simulink model "EcoSIM3_P2_C2_WIP"  (R2014b)
settings: Solver=ode1  SolverMode=SingleTasking  StartTime=0.0  StopTime=4  FixedStep=0.01  RelTol=1e-3
PostLoadFcn:
  | %, if any(exist('dsrtsu_mdlpostloadfcn', 'file') == [2, 3, 6]), try dsrtsu_mdlpostloadfcn('Execute', bdroot); catch fprintf('Error in PostLoadFcn (dsrtsu_mdlpostloadfcn) for model "%s":\n %s\n', bdroot, lasterr); end, end,
InitFcn:
  | tic
  | %Startup_EcoSIM
undefined symbols (not defined in the file or in its folder): canChannel, Controls, DriveCycles, Driver, EM_EFF_MAP, EM_PwrLoss_MAP, EngPwr, EngSpd, EngTrq, Glbl, Overwritten_Mode, Plants, Power, sigbuilder_block, Torque, Trialmap, Veh_Dynamics
libraries: simulink x135, canmsglib x113, fl_lib x104, canlib x89, nesl_utility x56, sdl_lib x29, dspsigops x6, dspswit3 x5, dspstat3 x2, commnoisgen2 x1, dspfdesign x1
(part 2 of 21)

== system EcoSIM3_P2_C2_WIP/Powertrain/Vehicle Dynamics ==
  note: 0.34 - Dynamic Rolling radius that
      | Brandon has for Goodyear Eagle tyres
  note: Tyre diameter- If tyre dia is kept at dyno test value (original * 1.12), energy consumption
      | for drive cycles is low as motor speed decreases, but time taken to reach 60 mph
      | increases because road torque decreases
  note: Velocity of the vehicle in m/s
  note: VEHICLE DYNAMICS
  note: Negative Torque from brakes
  Beta : Inport
  " Front Right Tire" : sdl_lib/Tires & Vehicles/Tire (Magic Formula)  parameterization=1  F_z1=Plants.Front_wh.Rated_Vertical_Load N  F_x1=Plants.Front_wh.Rated_Peak_Long_Force N  kappa1=Plants.Front_wh.Tire.Slip_At_Peak_Force  B_m=10  C_m=1.9  D_m=1  E_m=0.97  fz0=4e+3 N  p_Cx=1.685  p_Dx=[ 1.21 -0.037 ]  p_Ex=[ 0.344 0.095 -0.02 0 ]  p_Kx=[ 21.51 -0.163 0.245 ]  p_Hx=[ -0.002 0.002 ]  p_Vx=[ 0 0 ]  v_tr_thr=Plants.Front_wh.Tire.Slip_Calculation_Velocity_Threshold m/s  r_e=Plants.Front_wh.Tire.rollrad m  model_compliance=0  stiffness=1e+6 N/m  damping=1000 N/(m/s)  model_inertia=1  inertia=Plants.Front_wh.Wheel_Inertia kg*m^2  initial_velocity=0 rpm  model_resistance=1  resistance_model=1  coeff=Plants.Front_wh.Tire.Constant_coeff  p_tire=250e3 Pa  alpha=-0.003  beta=0.97  coeff_a=84e-4  coeff_b=6.2e-4 s/m  coeff_c=1.6e-4 s^2/m^2  v_thr=Plants.Front_wh.Tire.Velocity_threshold m/s
  1-D Lookup Table : Lookup_n-D  NumberOfTableDimensions=1  BreakpointsForDimension1=Plants.Front_br.Brake_Beta_Cmd  Table=Plants.Front_br.Brake_Friction_Map  InternalRulePriority=Speed  RndMeth=Simplest  InputSameDT=on
  Double-Shoe Brake1 : sdl_lib/Brakes & Detents/Rotational/Double-Shoe Brake  r_drum=Plants.Front_br.Drum_radius mm  r_act=Plants.Front_br.Actuator_location mm  r_pin=Plants.Front_br.Pin_location_rad mm  theta_pin=Plants.Front_br.Pin_location_ang deg  theta_0=Plants.Front_br.Shoe_begin_ang deg  theta_shoe=Plants.Front_br.Shoe_span deg  mu_visc=Plants.Front_br.Viscous_fric_coeff N*m/(rad/s)  mu=Plants.Front_br.Contact_fric_coeff  w_thr=Plants.Front_br.Angular_vel_threshold rad/s
  Double-Shoe Brake2 : sdl_lib/Brakes & Detents/Rotational/Double-Shoe Brake  r_drum=Plants.Rear_br.Drum_radius mm  r_act=Plants.Rear_br.Actuator_location mm  r_pin=Plants.Rear_br.Pin_location_rad mm  theta_pin=Plants.Rear_br.Pin_location_ang deg  theta_0=Plants.Rear_br.Shoe_begin_ang deg  theta_shoe=Plants.Rear_br.Shoe_span deg  mu_visc=Plants.Rear_br.Viscous_fric_coeff N*m/(rad/s)  mu=Plants.Rear_br.Contact_fric_coeff  w_thr=Plants.Rear_br.Angular_vel_threshold rad/s
  Double-Shoe Brake3 : sdl_lib/Brakes & Detents/Rotational/Double-Shoe Brake  r_drum=Plants.Front_br.Drum_radius mm  r_act=Plants.Front_br.Actuator_location mm  r_pin=Plants.Front_br.Pin_location_rad mm  theta_pin=Plants.Front_br.Pin_location_ang deg  theta_0=Plants.Front_br.Shoe_begin_ang deg  theta_shoe=Plants.Front_br.Shoe_span deg  mu_visc=Plants.Front_br.Viscous_fric_coeff N*m/(rad/s)  mu=Plants.Front_br.Contact_fric_coeff  w_thr=Plants.Front_br.Angular_vel_threshold rad/s
  Double-Shoe Brake4 : sdl_lib/Brakes & Detents/Rotational/Double-Shoe Brake  r_drum=Plants.Rear_br.Drum_radius mm  r_act=Plants.Rear_br.Actuator_location mm  r_pin=Plants.Rear_br.Pin_location_rad mm  theta_pin=Plants.Rear_br.Pin_location_ang deg  theta_0=Plants.Rear_br.Shoe_begin_ang deg  theta_shoe=Plants.Rear_br.Shoe_span deg  mu_visc=Plants.Rear_br.Viscous_fric_coeff N*m/(rad/s)  mu=Plants.Rear_br.Contact_fric_coeff  w_thr=Plants.Rear_br.Angular_vel_threshold rad/s
  Front Brake Bias : fl_lib/Physical Signals/Functions/PS Gain  gain=Plants.Front_br.brake_F_propor
  Front Left Tire : sdl_lib/Tires & Vehicles/Tire (Magic Formula)  parameterization=1  F_z1=Plants.Front_wh.Rated_Vertical_Load N  F_x1=Plants.Front_wh.Rated_Peak_Long_Force N  kappa1=Plants.Front_wh.Tire.Slip_At_Peak_Force  B_m=10  C_m=1.9  D_m=1  E_m=0.97  fz0=4e+3 N  p_Cx=1.685  p_Dx=[ 1.21 -0.037 ]  p_Ex=[ 0.344 0.095 -0.02 0 ]  p_Kx=[ 21.51 -0.163 0.245 ]  p_Hx=[ -0.002 0.002 ]  p_Vx=[ 0 0 ]  v_tr_thr=Plants.Front_wh.Tire.Slip_Calculation_Velocity_Threshold m/s  r_e=Plants.Front_wh.Tire.rollrad m  model_compliance=0  stiffness=1e+6 N/m  damping=1000 N/(m/s)  model_inertia=1  inertia=Plants.Front_wh.Wheel_Inertia kg*m^2  initial_velocity=0 rpm  model_resistance=1  resistance_model=1  coeff=Plants.Front_wh.Tire.Constant_coeff  p_tire=250e3 Pa  alpha=-0.003  beta=0.97  coeff_a=84e-4  coeff_b=6.2e-4 s/m  coeff_c=1.6e-4 s^2/m^2  v_thr=Plants.Front_wh.Tire.Velocity_threshold m/s
  PS-Simulink Converter : nesl_utility/PS-Simulink Converter  PhysicalDomain=network_engine_domain  SubClassName=ps_output  LeftPortType=input  RightPortType=output  PseudoPeriodic=off  Frequencies=[]  Unit=1  AffineConversion=off
  PS-Simulink Converter1 : nesl_utility/PS-Simulink Converter  PhysicalDomain=network_engine_domain  SubClassName=ps_output  LeftPortType=input  RightPortType=output  PseudoPeriodic=off  Frequencies=[]  Unit=1  AffineConversion=off
  Rear Differential : sdl_lib/Gears/Differential  driveshaft_location=2  cd_ratio=Plants.Rear_Diff.Diff_ratio  friction_model=2  efficiency=Plants.Rear_Diff.Ordinary_efficiencies  mu_visc=Plants.Rear_Diff.damp N*m/(rad/s)  w_thr=Plants.Rear_Diff.Velocity_thresholds rad/s
  Rear Brake Bias : fl_lib/Physical Signals/Functions/PS Gain  gain=Plants.Rear_br.brake_R_propor
  Rear Right Tire : sdl_lib/Tires & Vehicles/Tire (Magic Formula)  parameterization=1  F_z1=Plants.Rear_wh.Rated_Vertical_Load N  F_x1=Plants.Rear_wh.Rated_Peak_Long_Force N  kappa1=Plants.Rear_wh.Tire.Slip_At_Peak_Force  B_m=10  C_m=1.9  D_m=1  E_m=0.97  fz0=4e+3 N  p_Cx=1.685  p_Dx=[ 1.21 -0.037 ]  p_Ex=[ 0.344 0.095 -0.02 0 ]  p_Kx=[ 21.51 -0.163 0.245 ]  p_Hx=[ -0.002 0.002 ]  p_Vx=[ 0 0 ]  v_tr_thr=Plants.Rear_wh.Tire.Slip_Calculation_Velocity_Threshold m/s  r_e=Plants.Front_wh.Tire.rollrad m  model_compliance=0  stiffness=1e+6 N/m  damping=1000 N/(m/s)  model_inertia=1  inertia=Plants.Rear_wh.Wheel_Inertia kg*m^2  initial_velocity=0 rpm  model_resistance=1  resistance_model=1  coeff=Plants.Rear_wh.Tire.Constant_coeff  p_tire=250e3 Pa  alpha=-0.003  beta=0.97  coeff_a=84e-4  coeff_b=6.2e-4 s/m  coeff_c=1.6e-4 s^2/m^2  v_thr=Plants.Rear_wh.Tire.Velocity_threshold m/s
  Rear Right Tires : sdl_lib/Tires & Vehicles/Tire (Magic Formula)  parameterization=1  F_z1=Plants.Rear_wh.Rated_Vertical_Load N  F_x1=Plants.Rear_wh.Rated_Peak_Long_Force N  kappa1=Plants.Rear_wh.Tire.Slip_At_Peak_Force  B_m=10  C_m=1.9  D_m=1  E_m=0.97  fz0=4e+3 N  p_Cx=1.685  p_Dx=[ 1.21 -0.037 ]  p_Ex=[ 0.344 0.095 -0.02 0 ]  p_Kx=[ 21.51 -0.163 0.245 ]  p_Hx=[ -0.002 0.002 ]  p_Vx=[ 0 0 ]  v_tr_thr=Plants.Rear_wh.Tire.Slip_Calculation_Velocity_Threshold m/s  r_e=Plants.Front_wh.Tire.rollrad m  model_compliance=0  stiffness=1e+6 N/m  damping=1000 N/(m/s)  model_inertia=1  inertia=Plants.Rear_wh.Wheel_Inertia kg*m^2  initial_velocity=0 rpm  model_resistance=1  resistance_model=1  coeff=Plants.Rear_wh.Tire.Constant_coeff  p_tire=250e3 Pa  alpha=-0.003  beta=0.97  coeff_a=84e-4  coeff_b=6.2e-4 s/m  coeff_c=1.6e-4 s^2/m^2  v_thr=Plants.Rear_wh.Tire.Velocity_threshold m/s
  Road Grade : fl_lib/Physical Signals/Sources/PS Constant  constant=0
  Scope1 : Scope  Commented=on  NumInputPorts=2
      settings: TimeRange=0.05746676406135975  YMin=-0.001119~-0.000858  YMax=-0.00111~-0.00084  SaveName=ScopeData11
  Sensor : Subsystem
  Simulink-PS Converter1 : nesl_utility/Simulink-PS Converter  PhysicalDomain=network_engine_domain  SubClassName=ps_input  LeftPortType=input  RightPortType=output  PseudoPeriodic=off  Frequencies=[]  NoiseDistribution=none  NoiseParameters=[]  Unit=N  AffineConversion=off  InputFiltering=off  SimscapeFilterOrder=1  InputFilterTimeConstant=0.001  UdotUserProvided=1
  Subsystem : Subsystem
  Vehicle Body : sdl_lib/Tires & Vehicles/Vehicle Body  mass=Veh_Dynamics.Body.Mass kg  n_w=2  x_f=Veh_Dynamics.Body.Distance_CG_FrontAxle m  x_r=Veh_Dynamics.Body.Distance_CG_RearAxle m  y_c=Veh_Dynamics.Body.Distance_CG_Ground m  area=Veh_Dynamics.Body.Frontal_Area m^2  Cd=Veh_Dynamics.Body.Aero_Drag_Coeff  v0=0 m/s  g=9.81 m/s^2  rho=1.18 kg/m^3
  Wind velocity : fl_lib/Physical Signals/Sources/PS Constant  constant=0
  MC_Coupler_Out : PMIOPort  Tag=PMCPort  Port=1  Side=Left
  Vehicle_Speed [m/s] : Outport
  wires:
  PS-Simulink Converter/1 -> Scope1/1  "LF_Wheel_Slip"
  PS-Simulink Converter1/1 -> Scope1/2  "LR_Wheel_Slip"
  Beta/1 -> 1-D Lookup Table/1
  1-D Lookup Table/1 -> Simulink-PS Converter1/1
  Sensor/1(Sensor_Out) -> Vehicle_Speed [m/s]/1
  connections:
  " Front Right Tire"/LConn1 -- Vehicle Body/RConn2 -- Front Left Tire/LConn1
  Rear Right Tire/LConn1 -- Vehicle Body/RConn1 -- Rear Right Tires/LConn1
  Sensor/RConn1 -- Rear Differential/RConn2 -- Rear Right Tires/LConn2 -- Double-Shoe Brake2/LConn2
  Rear Right Tire/LConn2 -- Double-Shoe Brake4/LConn2 -- Sensor/RConn2 -- Rear Differential/RConn1
  " Front Right Tire"/RConn2 -- Front Left Tire/RConn2 -- Subsystem/RConn1 -- Rear Right Tire/RConn2 -- Rear Right Tires/RConn2
  Rear Brake Bias/LConn1 -- Simulink-PS Converter1/RConn1 -- Front Brake Bias/LConn1
  Double-Shoe Brake3/LConn1 -- Double-Shoe Brake1/LConn1 -- Front Brake Bias/RConn1
  Front Left Tire/LConn2 -- Sensor/LConn3 -- " Front Right Tire"/LConn2 -- Sensor/LConn2 -- Double-Shoe Brake1/LConn2 -- Double-Shoe Brake3/LConn2
  Double-Shoe Brake2/LConn1 -- Rear Brake Bias/RConn1 -- Double-Shoe Brake4/LConn1
  Subsystem/LConn1 -- Vehicle Body/LConn1
  Road Grade/RConn1 -- Vehicle Body/RConn3
  PS-Simulink Converter1/LConn1 -- Rear Right Tires/RConn1
  PS-Simulink Converter/LConn1 -- " Front Right Tire"/RConn1
  Vehicle Body/LConn2 -- Sensor/LConn1
  MC_Coupler_Out/RConn1 -- Rear Differential/LConn1
  Vehicle Body/LConn3 -- Wind velocity/RConn1

== system EcoSIM3_P2_C2_WIP/RTI Data/RTI Data Store ==
  RTI Data Store : Subsystem  mask(RTI_DATA_STORE){}
      mask help:
      | RTI Data Store Block. This block is used by RTI to store internal model dependent data. Deleting this block will result in data loss.
      |
      | NEVER DELETE, COPY, OR MODIFY THIS BLOCK!
      mask Help:
      | RTI Data Store Block. This block is used by RTI to store internal model dependent data. Deleting this block will result in data loss.
      | 
      | NEVER DELETE, COPY, OR MODIFY THIS BLOCK!
      mask Display: text(0.5, 0.5, ' ', 'HorizontalAlignment', 'center');

== system EcoSIM3_P2_C2_WIP/Supervisory Controller/Charging Handshake ==
  In1 : Inport
  Bus Creator : BusCreator  Inputs=2
  Bus Selector1 : BusSelector  OutputSignals=From_GCM.GCM_CAN_Out.charge_mode_request,ESS_Transmit.ESS_Electrical_Out.chga_ena,ESS_Transmit.ESS_CAN_Out.BCM_Status.bcm_chg_done,ESS_Transmit.ESS_CAN_Out.BCM_Data2.bcm_balancing,ESS_Transmit.ESS_CAN_Out.BCM_Status.bcm_ready,ESS_Transmit.ESS_CAN_Out.BCM_Status.bcm_on_plug,ESS_Transmit.ESS_CAN_Out.BCM_Status.bcm_chgc_stat
  Chart1 : Stateflow chart  TreatAsAtomicUnit=on
  Compare To Constant : simulink/Logic and Bit Operations/Compare To Constant  relop===  const=1  OutDataTypeStr=boolean
  Constant1 : Constant  Value=0
  Data Type Conversion : DataTypeConversion
  Data Type Conversion1 : DataTypeConversion
  Terminator1 : Terminator
  Terminator3 : Terminator
  Out1 : Outport
  tag scope: Charging_Complete=global
  wires:
  Data Type Conversion1/1 -> Bus Creator/2  "PON"
  Data Type Conversion/1 -> Bus Creator/1  "chga_wake"
  Bus Selector1/1 -> Chart1/1(charge_mode_request)  "<charge_mode_request>"
  Bus Selector1/2 -> Chart1/2(chga_ena)  "<chga_ena>"
  Chart1/1(chga_wake) -> Data Type Conversion/1
  Chart1/2(PON) -> Data Type Conversion1/1
  Bus Creator/1 -> Out1/1
  In1/1 -> Bus Selector1/1
  Constant1/1 -> Chart1/4(bcm_balancing)
  Bus Selector1/3 -> Chart1/3(bcm_chg_done)  "<bcm_chg_done>"
  Bus Selector1/4 -> Terminator1/1  "<bcm_balancing>"
  Chart1/3(Charging_Complete) -> [Charging_Complete]
  Bus Selector1/5 -> Chart1/5(bcm_ready)  "<bcm_ready>"
  Bus Selector1/6 -> Chart1/6(bcm_on_plug)  "<bcm_on_plug>"
  Bus Selector1/7 -> Compare To Constant/1  "<bcm_chgc_stat>"
  Compare To Constant/1 -> Terminator3/1  "Charging_Light_On"

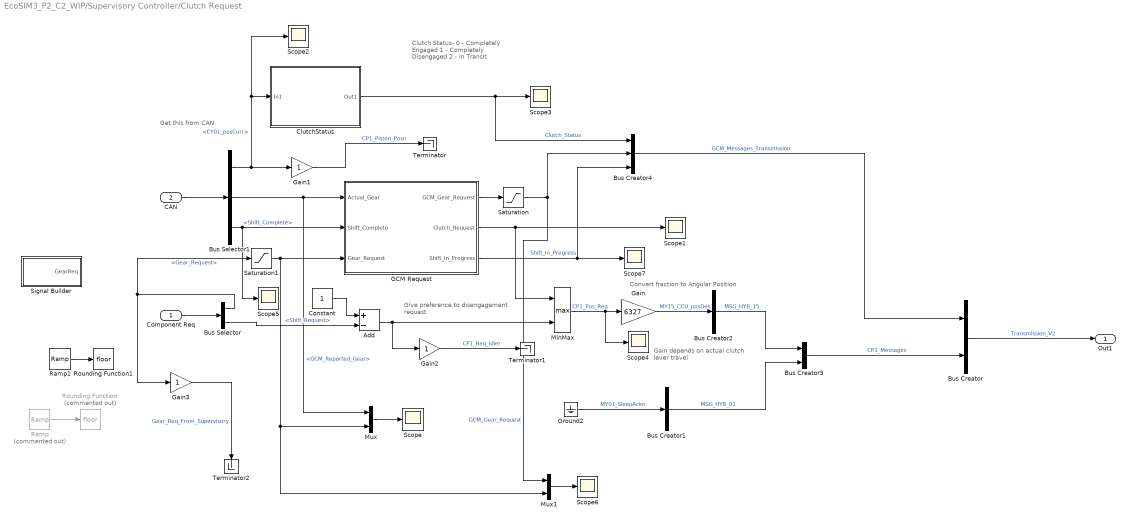
== system EcoSIM3_P2_C2_WIP/Supervisory Controller/Clutch Request ==
  note: Get this from CAN
  note: Convert fraction to Angular Position
  note: Clutch Status-
      | 0 - Completely Engaged
      | 1 - Completely Disengaged
      | 2 - In Transit
  note: Gain depends on actual
      | clutch lever travel
  note: Give preference to disengagement
      | request
  Component Req : Inport
  CAN : Inport  Port=2
  Add : Sum  Inputs=+-
  Bus Creator : BusCreator  Inputs=2
  Bus Creator1 : BusCreator  Inputs=1
  Bus Creator2 : BusCreator  Inputs=1
  Bus Creator3 : BusCreator  Inputs=2
  Bus Creator4 : BusCreator  Inputs=3
  Bus Selector : BusSelector  OutputSignals=Trans_Receive.Gear_Request,Trans_Receive.Shift_Request
  Bus Selector1 : BusSelector  OutputSignals=CP1_Transmit.CP1_CAN_Out.CCU_HYB_01.CY01_posCurr,From_GCM.GCM_CAN_Out.Shift_Status_to_MABx.GCM_Reported_Gear,From_GCM.GCM_CAN_Out.Shift_Status_to_MABx.Shift_Complete
  ClutchStatus : Subsystem
  Constant : Constant
  GCM Request : Stateflow chart  TreatAsAtomicUnit=on
  Gain : Gain  Gain=6327
  Gain1 : Gain
  Gain2 : Gain
  Gain3 : Gain
  Ground2 : Ground
  MinMax : MinMax  Function=max  Inputs=2
  Mux : Mux  Inputs=2
  Mux1 : Mux  Inputs=2
  Ramp : simulink/Sources/Ramp  Commented=on  slope=1  start=0  X0=1
  Ramp1 : simulink/Sources/Ramp  slope=0.5  start=0  X0=-1
  Rounding Function : Rounding  Commented=on
  Rounding Function1 : Rounding
  Saturation : Saturate  UpperLimit=5  LowerLimit=-1
  Saturation1 : Saturate  UpperLimit=5  LowerLimit=-1
  Scope{,1..7} (8 alike) : Scope
      Scope settings: YMin=0  SaveName=ScopeData20
      Scope1 settings: SaveName=ScopeData22
      Scope2 settings: YMin=0  YMax=8000  SaveName=ScopeData35
      Scope3 settings: YMin=0  YMax=8000  SaveName=ScopeData36
      Scope4 settings: SaveName=ScopeData37
      Scope5 settings: SaveName=ScopeData38
      Scope6 settings: SaveName=ScopeData45
      Scope7 settings: SaveName=ScopeData61
  Signal Builder : Subsystem  Tag=STV Subsys  LoadFcn=sigbuilder_block('load');  StartFcn=sigbuilder_block('start');  StopFcn=sigbuilder_block('stop');  ClipboardFcn=sigbuilder_block('clipboard');  mask(Sigbuilder block){}
      mask help: Simulink:masks:SigbuilderBlock_MD
      mask init:
      | if ~strcmp(get_param(bdroot(gcbh),'SimulationStatus'),'stopped') tuvar = sigbuilder_block('maskInit'); end
      settings: CopyFcn=sigbuilder_block('copy');  DeleteFcn=sigbuilder_block('delete');  ModelCloseFcn=sigbuilder_block('modelClose');  PreSaveFcn=sigbuilder_block('preSave');  PauseFcn=sigbuilder_block('pause');  ContinueFcn=sigbuilder_block('continue');  NameChangeFcn=sigbuilder_block('namechange');  OpenFcn=sigbuilder_block('open',[437.6 199.2 550.4 400 ]);  CloseFcn=sigbuilder_block('close');
      mask Display: plot(0, 0, 100, 100,[2, 2, 32, 32, 2], [68, 8, 8, 68, 68],[32, 2], [38, 38], [32, 19, 2],[53, 60, 44], [32, 17, 17, 2],[16, 16, 31, 31]);txt = getActiveGroup(gcbh);text(2, 100, txt,'verticalAlignment', 'top');
  Terminator : Terminator
  Terminator1 : Terminator
  Terminator2 : Terminator
  Out1 : Outport
  wires:
  Component Req/1 -> Bus Selector/1
  CAN/1 -> Bus Selector1/1
  Bus Selector1/2 -> GCM Request/1(Actual_Gear), Mux/1  "<GCM_Reported_Gear>"
  Bus Selector/1 -> Gain3/1, Saturation1/1  "<Gear_Request>"
  GCM Request/2(Clutch_Request) -> MinMax/1, Scope1/1
  MinMax/1 -> Scope4/1, Gain/1  "CP1_Pos_Req"
  Ground2/1 -> Bus Creator1/1  "MY01_SleepAckn"
  Gain/1 -> Bus Creator2/1  "MY15_CCU_posDes"
  Bus Creator2/1 -> Bus Creator3/1  "MSG_HYB_15"
  Bus Creator1/1 -> Bus Creator3/2  "MSG_HYB_01"
  Bus Creator3/1 -> Bus Creator/2  "CP1_Messages"
  ClutchStatus/1(Out1) -> Scope3/1, Bus Creator4/1  "Clutch_Status"
  Saturation/1 -> Mux1/1, Bus Creator4/2  "GCM_Gear_Request"
  Bus Creator4/1 -> Bus Creator/1  "GCM_Messages_Transmission"
  Bus Creator/1 -> Out1/1  "Transmission_V2"
  Bus Selector1/3 -> Scope5/1, GCM Request/2(Shift_Complete)  "<Shift_Complete>"
  Bus Selector1/1 -> Gain1/1, Scope2/1, ClutchStatus/1(In1)  "<CY01_posCurr>"
  Mux/1 -> Scope/1
  GCM Request/1(GCM_Gear_Request) -> Saturation/1
  Gain1/1 -> Terminator/1  "CP1_Piston_Posn"
  Gain2/1 -> Terminator1/1  "CP1_Req_Idler"
  Bus Selector/2 -> Add/2  "<Shift_Request>"
  Constant/1 -> Add/1
  Add/1 -> MinMax/2, Gain2/1
  Saturation1/1 -> Mux1/2, Mux/2, GCM Request/3(Gear_Request)
  Ramp/1 -> Rounding Function/1
  Mux1/1 -> Scope6/1
  Ramp1/1 -> Rounding Function1/1
  Gain3/1 -> Terminator2/1  "Gear_Req_From_Supervisory"
  GCM Request/3(Shift_In_Progress) -> Scope7/1, Bus Creator4/3  "Shift_In_Progress"

== system EcoSIM3_P2_C2_WIP/Supervisory Controller/Driver Requested Torque ==
  CAN IN : Inport
  Add : Sum
  Bias : Bias  Bias=-1
  Bias1 : Bias  Bias=1
  Bus Selector : BusSelector  OutputSignals=From_GCM.GCM_CAN_Out.Shift_Status_to_MABx.GCM_Reported_Gear,Vehicle_speed.Vehicle_Speed_meter_per_s,From_GCM.GCM_CAN_Out.Shift_Status_to_MABx.GCM_Reported_Gear,ModeSwitch_Conditioned.DRIV_mode,Alpha_percent
  Constant : Constant  Value=0
  Display : Display
  EM Max Torque : Lookup_n-D  BreakpointsForDimension1=Plants.EM.Mdl.Plant.max_min_RPM  BreakpointsForDimension2=[0,1]  Table=[Plants.EM.Mdl.Plant.T_max_Cont',Plants.EM.Mdl.Plant.T_max_Peak']  InternalRulePriority=Speed  RndMeth=Simplest  InputSameDT=on
  Max Torque Calculation : Subsystem
  Memory13 : Memory  X0=1
  PTU Ratio : Gain  Gain=2.77*2.77
  Pedal Map : Lookup_n-D  BreakpointsForDimension1=[0 100]  BreakpointsForDimension2=[2,3]  Table=[0 0;2000 4000]  InternalRulePriority=Speed  RndMeth=Simplest  InputSameDT=on
  Saturation Dynamic : simulink/Discontinuities/Saturation Dynamic  OutMin=[]  OutMax=[]  OutDataTypeStr=Inherit: Same as second input  OutDataType=fixdt(1, 16)  OutScaling=2^-10  DoSatur=off
  Scope : Scope
      settings: SaveName=ScopeData68
  Scope1 : Scope
      settings: SaveName=ScopeData70
  Speed Calculations : Subsystem
  Driver Torque Request : Outport
  wires:
  Bus Selector/5 -> Pedal Map/1  "<Alpha_percent>"
  Pedal Map/1 -> Saturation Dynamic/2  "Driver Torque Request"
  Saturation Dynamic/1 -> Driver Torque Request/1  "Driver Torque Request"
  Constant/1 -> Saturation Dynamic/3
  Speed Calculations/1(Engine Speed) -> Max Torque Calculation/2(Engine Speed)
  Max Torque Calculation/1("Engine Torque ") -> Add/1
  EM Max Torque/1 -> Scope1/1, PTU Ratio/1
  Speed Calculations/2("EM Speed ") -> EM Max Torque/1
  PTU Ratio/1 -> Add/2
  CAN IN/1 -> Bus Selector/1
  Bus Selector/2 -> Speed Calculations/1("Vehicle Speed m/s ")  "<Vehicle_Speed_meter_per_s>"
  Memory13/1 -> Speed Calculations/2(Gear Current)
  Bus Selector/3 -> Memory13/1  "<GCM_Reported_Gear>"
  Bus Selector/1 -> Max Torque Calculation/1(Gear)  "<GCM_Reported_Gear>"
  Bias1/1 -> Pedal Map/2
  Bias/1 -> EM Max Torque/2
  Bus Selector/4 -> Bias1/1, Bias/1  "<DRIV_mode>"
  Add/1 -> Saturation Dynamic/1, Scope/1, Display/1

== system EcoSIM3_P2_C2_WIP/Supervisory Controller/Functional Safety1 ==
  CAN Inputs : Inport
  Functional Safety Algorithm : Subsystem
  Terminator : Terminator
  Out1 : Outport
  wires:
  CAN Inputs/1 -> Functional Safety Algorithm/2(ECU/Sensor Signals), Functional Safety Algorithm/1(Torque Requests)  "CAN_Inputs"
  Functional Safety Algorithm/2(Fault Code) -> Out1/1  "Fault_Code"
  Functional Safety Algorithm/1(Torque Limits) -> Terminator/1  "Torque_Limits"

== system EcoSIM3_P2_C2_WIP/Supervisory Controller/Input Conditioning ==
  note: In here I would like to pull off the signals that I actually need from each message
  Raw Signals : Inport
  Alpha Conditioning : Subsystem
  Bus Creator : BusCreator  Inputs=11
  Bus Selector : BusSelector  OutputSignals=ESS_Transmit,EM_Transmit,ICE_Transmit,BAS_Transmit,From_GCM,GM_Transmit,CP1_Transmit
  ModeSwitch Conditioning : Subsystem
  PRNDL Conditioning : Subsystem
  Velocity Conditioning : Subsystem
  Conditioned Signals : Outport
  wires:
  Bus Creator/1 -> Conditioned Signals/1
  Alpha Conditioning/1(Alpha Percent) -> Bus Creator/3
  Velocity Conditioning/1(Velocity Processed) -> Bus Creator/4
  Raw Signals/1 -> Bus Selector/1, Velocity Conditioning/1(Raw Ticks), Alpha Conditioning/1(Raw Alpha_V), PRNDL Conditioning/1(PRNDL)
  Bus Selector/1 -> Bus Creator/5  "<ESS_Transmit>"
  Bus Selector/2 -> Bus Creator/6  "<EM_Transmit>"
  Bus Selector/3 -> Bus Creator/7  "<ICE_Transmit>"
  Bus Selector/4 -> Bus Creator/8  "<BAS_Transmit>"
  Bus Selector/5 -> Bus Creator/9  "<From_GCM>"
  Bus Selector/6 -> Bus Creator/10  "<GM_Transmit>"
  Bus Selector/7 -> Bus Creator/11  "<CP1_Transmit>"
  PRNDL Conditioning/1(Out1) -> Bus Creator/2
  ModeSwitch Conditioning/1(Out1) -> Bus Creator/1

== system EcoSIM3_P2_C2_WIP/Supervisory Controller/Mode Operation ==
  Supervisory : Inport
  From CAN : Inport  Port=2
  Accessory : Subsystem
  Bus Selector : BusSelector  OutputSignals=Mode
  Charging : Subsystem
  Compare To Constant1 : simulink/Logic and Bit Operations/Compare To Constant  relop===  const=2  OutDataTypeStr=boolean
  Compare To Constant2 : simulink/Logic and Bit Operations/Compare To Constant  relop===  const=5  OutDataTypeStr=boolean
  Compare To Constant3 : simulink/Logic and Bit Operations/Compare To Constant  relop===  const=6  OutDataTypeStr=boolean
  Compare To Constant4 : simulink/Logic and Bit Operations/Compare To Constant  relop===  const=1  OutDataTypeStr=boolean
  Compare To Constant5 : simulink/Logic and Bit Operations/Compare To Constant  relop===  const=7  OutDataTypeStr=boolean
  Compare To Constant6 : simulink/Logic and Bit Operations/Compare To Constant  relop===  const=3  OutDataTypeStr=boolean
  Compare To Constant7 : simulink/Logic and Bit Operations/Compare To Constant  relop===  const=4  OutDataTypeStr=boolean
  Compare To Constant8 : simulink/Logic and Bit Operations/Compare To Constant  relop===  const=8  OutDataTypeStr=boolean
  Compare To Constant9 : simulink/Logic and Bit Operations/Compare To Constant  relop===  const=9  OutDataTypeStr=boolean
  EV : Subsystem
  "Engine Only " : Subsystem
  "Engine Start " : Subsystem
  From CAN{1..8} (8 alike) : InportShadow  Port=2
  Limited EV : Subsystem
  Multiport Switch : MultiPortSwitch  Inputs=9
  Saturation : Saturate  UpperLimit=9  LowerLimit=1
  Series : Subsystem  Commented=on
  Series1 : Subsystem
  Shutdown : Subsystem
  Startup : Subsystem
  Component Torque Request : Outport
  wires:
  Compare To Constant1/1 -> EV/Enable
  Compare To Constant5/1 -> Accessory/Enable
  Compare To Constant2/1 -> Limited EV/Enable
  Compare To Constant3/1 -> Shutdown/Enable
  Supervisory/1 -> Bus Selector/1, Startup/2("Supervisory "), Series1/2("Supervisory "), Charging/2("Supervisory "), Accessory/1("Supervisory "), Shutdown/2("Supervisory "), Limited EV/1("Supervisory "), "Engine Start "/1("Supervisory "), "Engine Only "/1("Supervisory "), EV/1("Supervisory ")
  From CAN/1 -> Shutdown/1(From CAN)
  From CAN1/1 -> Startup/1(From CAN)
  From CAN2/1 -> "Engine Only "/2(From CAN)
  Compare To Constant4/1 -> Startup/Enable
  Bus Selector/1 -> Saturation/1  "<Mode>"
  Compare To Constant6/1 -> "Engine Only "/Enable
  Compare To Constant7/1 -> "Engine Start "/Enable
  Compare To Constant8/1 -> Charging/Enable
  From CAN5/1 -> Charging/1(From CAN)
  From CAN3/1 -> Limited EV/2(CAN)
  From CAN7/1 -> EV/2(CAN)
  From CAN4/1 -> "Engine Start "/2("CAN In ")
  Multiport Switch/1 -> Component Torque Request/1
  Saturation/1 -> Multiport Switch/1, Compare To Constant4/1, Compare To Constant2/1, Compare To Constant9/1, Compare To Constant8/1, Compare To Constant5/1, Compare To Constant3/1, Compare To Constant7/1, Compare To Constant6/1, Compare To Constant1/1
  From CAN6/1 -> Accessory/2(CAN)
  Startup/1(Output) -> Multiport Switch/2
  EV/1(Output) -> Multiport Switch/3
  "Engine Only "/1("Output ") -> Multiport Switch/4
  "Engine Start "/1("Output ") -> Multiport Switch/5
  Limited EV/1(Output) -> Multiport Switch/6
  Shutdown/1(Output) -> Multiport Switch/7
  Accessory/1(Output) -> Multiport Switch/8
  Charging/1(Output) -> Multiport Switch/9
  Compare To Constant9/1 -> Series1/Enable
  From CAN8/1 -> Series1/1(From CAN)
  Series1/1("Output ") -> Multiport Switch/10

== system EcoSIM3_P2_C2_WIP/Supervisory Controller/Mode Selection  ==
  CAN IN : Inport
  "Fault_Code " : Inport  Port=2
  Startup : Inport  Port=3
  AllowStartStop : Constant  Value=0
  Bus Selector : BusSelector  OutputSignals=Vehicle_speed.Vehicle_Speed_meter_per_s,ESS_Transmit.ESS_CAN_Out.BCM_Status.bcm_soc,GM_Transmit.GMLAN_CAN_Out.PPEI_Brake_Apply_Status.BrkPdlPos,GM_Transmit.GMLAN_CAN_Out.PPEI_Platform_General_Status.SysPwrMd,ESS_Transmit.ESS_CAN_Out.BCM_Status.bcm_on_plug
  Bus Selector1 : BusSelector  OutputSignals=ICE_Request.Engine_On,ICE_Request.Engine_Run,Vehicle_Ready
  CAN IN1 : InportShadow
  Compare To Constant : simulink/Logic and Bit Operations/Compare To Constant  relop===  const=1  OutDataTypeStr=boolean
  Compare To Zero : simulink/Logic and Bit Operations/Compare To Zero  relop=<  OutDataTypeStr=boolean
  Constant : Constant  Commented=on  Value=2
  Constant1 : Constant  Value=0
  Constant3 : Constant  Value=0
  Data Type Conversion : DataTypeConversion
  Data Type Conversion1 : DataTypeConversion
  Display : Display
  Display1 : Display
  "Limp Home Mode Selection  " : Subsystem
  Logical Operator : Logic  AllPortsSameDT=off  OutDataTypeStr=boolean
  Memory : Memory
  Memory1 : Memory
  Memory2 : Memory
  Min_SOC : Constant  Value=18
  Mode Overide : Switch  Criteria=u2 > Threshold  Threshold=0.5
  "Mode Selection " : Stateflow chart  TreatAsAtomicUnit=on
  Product : Product
  Start-Stop control : Subsystem
  Startup1 : InportShadow  Port=3
  Step : Step  Commented=on  Time=20  After=0  SampleTime=0
  Mode Transmit : Outport
  wires:
  "Mode Selection "/1(VEH_Mode) -> "Limp Home Mode Selection  "/1("Mode Requested  ")
  Bus Selector/3 -> "Mode Selection "/4(beta)  "<BrkPdlPos>"
  Min_SOC/1 -> "Mode Selection "/3(Min_SOC)
  Constant3/1 -> "Mode Selection "/8(cs_switch)
  Bus Selector/4 -> Display/1, "Mode Selection "/5(SysPwrMd)  "<SysPwrMd>"
  Bus Selector/2 -> "Mode Selection "/2(SOC)  "<bcm_soc>"
  "Fault_Code "/1 -> "Limp Home Mode Selection  "/2("Fault Code ")  "hsc_FS_Fault_Code"
  CAN IN/1 -> Bus Selector/1
  Bus Selector/1 -> "Mode Selection "/1(Veh_Spd)  "<Vehicle_Speed_meter_per_s>"
  "Limp Home Mode Selection  "/1(Vehicle Mode) -> Mode Overide/3  "Mode"
  Compare To Zero/1 -> "Mode Selection "/10(Shutdown_Complete)
  Mode Overide/1 -> Mode Transmit/1
  Bus Selector/5 -> "Mode Selection "/11(bcm_on_plug), Display1/1  "<bcm_on_plug>"
  Startup/1 -> Bus Selector1/1
  Memory/1 -> Compare To Zero/1, Compare To Constant/1, "Mode Selection "/9(Vehicle_Ready)  "Vehicle_Ready"
  Bus Selector1/3 -> Memory/1  "<Vehicle_Ready>"
  Bus Selector1/2 -> Memory1/1  "<Engine_Run>"
  Bus Selector1/1 -> Memory2/1  "<Engine_On>"
  Memory2/1 -> Logical Operator/1
  Memory1/1 -> Logical Operator/2
  Logical Operator/1 -> Data Type Conversion/1
  Data Type Conversion/1 -> "Mode Selection "/6(eng_on)
  Constant1/1 -> "Mode Selection "/7(eng_switch)
  CAN IN1/1 -> Start-Stop control/1(From_CAN)
  Startup1/1 -> Start-Stop control/2(Startup)
  Start-Stop control/1(Mode) -> Mode Overide/1
  AllowStartStop/1 -> Product/1
  Product/1 -> Mode Overide/2
  Compare To Constant/1 -> Data Type Conversion1/1
  Data Type Conversion1/1 -> Product/2

== system EcoSIM3_P2_C2_WIP/Supervisory Controller/Outout Conditioning ==
  NonProp : Inport
  In1 : Inport  Port=2
  CP1 : Inport  Port=3
  In2 : Inport  Port=4
  Bus Creator : BusCreator  Inputs=2
  Bus Creator1 : BusCreator  Inputs=2
  Bus Creator2 : BusCreator  Inputs=9
  Bus Selector : BusSelector  OutputSignals=PON,chga_wake
  Bus Selector1 : BusSelector  OutputSignals=ESS_Signals_A123,EM_Messages_Rhinehart,BAS_Infineon_Messages,Engine_Messages,Trans_Receive,Supervisory
  Bus Selector2 : BusSelector  OutputSignals=GCM_Messages_Transmission,CP1_Messages
  Bus Selector3 : BusSelector  OutputSignals=DC_DC
  Out1 : Outport
  wires:
  Bus Creator2/1 -> Bus Creator/1  "Supervisory_CAN"
  Bus Creator1/1 -> Bus Creator/2  "Supervisory_Electrical"
  Bus Creator/1 -> Out1/1  "Supervisory_Requests"
  In2/1 -> Bus Selector/1
  Bus Selector/1 -> Bus Creator1/1  "<PON>"
  Bus Selector/2 -> Bus Creator1/2  "<chga_wake>"
  In1/1 -> Bus Selector1/1  "Supervisory_CAN"
  CP1/1 -> Bus Selector2/1
  Bus Selector2/1 -> Bus Creator2/1  "<GCM_Messages_Transmission>"
  Bus Selector2/2 -> Bus Creator2/2  "<CP1_Messages>"
  Bus Selector1/3 -> Bus Creator2/5  "<BAS_Infineon_Messages>"
  Bus Selector1/2 -> Bus Creator2/4  "<EM_Messages_Rhinehart>"
  Bus Selector1/6 -> Bus Creator2/8  "<Supervisory>"
  Bus Selector1/4 -> Bus Creator2/6  "<Engine_Messages>"
  Bus Selector1/5 -> Bus Creator2/7  "<Trans_Receive>"
  Bus Selector1/1 -> Bus Creator2/3  "<ESS_Signals_A123>"
  NonProp/1 -> Bus Selector3/1
  Bus Selector3/1 -> Bus Creator2/9  "<DC_DC>"

== system EcoSIM3_P2_C2_WIP/Supervisory Controller/PRNDL ==
  note: need to include PRNDL Logic here
  Controller Inputs : Inport
  "From CAN " : Inport  Port=2
  Clutch : Inport  Port=3
  Compare To Constant : simulink/Logic and Bit Operations/Compare To Constant  relop===  const=1  OutDataTypeStr=boolean
  Compare To Constant1 : simulink/Logic and Bit Operations/Compare To Constant  relop===  const=2  OutDataTypeStr=boolean
  Compare To Constant2 : simulink/Logic and Bit Operations/Compare To Constant  relop===  const=3  OutDataTypeStr=boolean
  Compare To Constant3 : simulink/Logic and Bit Operations/Compare To Constant  relop===  const=4  OutDataTypeStr=boolean
  D : Constant  Commented=on  Value=4
  Determine Gear : Subsystem
  Determine Gear1 : Subsystem  Commented=on
  Display : Display
  Drive : Subsystem
  Memory : Memory  X0=1
  Multiport Switch : MultiPortSwitch  Inputs=4
  "Neutral " : Subsystem
  Park : Subsystem
  Reverse : Subsystem
  Saturation : Saturate  UpperLimit=4  LowerLimit=1
  Signal Conversion : SignalConversion
  "Total Torque " : Outport
  wires:
  Compare To Constant/1 -> Park/Enable
  Compare To Constant1/1 -> Reverse/Enable
  Compare To Constant2/1 -> "Neutral "/Enable
  Compare To Constant3/1 -> Drive/Enable
  Signal Conversion/1 -> "Total Torque "/1
  Controller Inputs/1 -> Drive/1(In1), "Neutral "/1(Treq), Reverse/1(Treq), Park/1(Treq), Determine Gear/2(HSC Inputs)
  Determine Gear/1(Gear) -> Saturation/1, Display/1
  Multiport Switch/1 -> Signal Conversion/1
  Drive/1(HSC_Out) -> Multiport Switch/5
  Saturation/1 -> Memory/1
  "Neutral "/1("HSC_Out ") -> Multiport Switch/4
  Reverse/1("HSC_Out ") -> Multiport Switch/3
  Park/1(HSC_Out) -> Multiport Switch/2
  Memory/1 -> Compare To Constant/1, Compare To Constant1/1, Compare To Constant2/1, Compare To Constant3/1, Multiport Switch/1
  "From CAN "/1 -> Drive/2(CAN), "Neutral "/2(CAN), Reverse/2(CAN), Park/2(CAN), Determine Gear/1(From CAN)
  Clutch/1 -> Drive/3(Clutch)

== system EcoSIM3_P2_C2_WIP/Supervisory Controller/Simple Fault Detection ==
  In1 : Inport
  Battery Shutdown : Constant  Value=58
  Bus Selector : BusSelector  OutputSignals=EM_Transmit.EM_CAN_Out.M162_Temperature_Set_3.Motor_Temperature,ESS_Transmit.ESS_CAN_Out.BCM_Data1.bcm_cell_tmax,EM_Transmit.EM_CAN_Out,ESS_Transmit.ESS_CAN_Out.BCM_Limits.bcm_dis_buf
  "CAN Communication Failures " : Subsystem
  Constant : Constant  Value=160
  Constant1 : Constant  Commented=on  Value=0
  Fault Code Determination : Stateflow chart  TreatAsAtomicUnit=on
  Ground : Ground
  Inverter Shutdown : Constant  Value=94
  "Inverter Temp Selection " : Subsystem
  Inverter Warning : Constant  Value=70
  Mode Overide : Switch  Criteria=u2 > Threshold
  Motor Shutdown : Constant  Value=150
  "Motor Warning " : Constant  Value=100
  Scope : Scope  NumInputPorts=3
      settings: TimeRange=240  YMin=-1~30~0  YMax=1~75~3
  Step : Step  Time=15  After=0  SampleTime=0
  Terminator : Terminator
  "Fault Code " : Outport
  wires:
  In1/1 -> Bus Selector/1
  Constant/1 -> Mode Overide/1
  Bus Selector/1 -> Mode Overide/3  "<Motor_Temperature>"
  Mode Overide/1 -> Fault Code Determination/1(EM_Temp)
  Battery Shutdown/1 -> Fault Code Determination/9(Battery_Shutdown)
  Inverter Shutdown/1 -> Fault Code Determination/7(Inverter_Shutdown)
  Inverter Warning/1 -> Fault Code Determination/6(Inverter_Warning)
  Motor Shutdown/1 -> Fault Code Determination/5(EM_Shutdown)
  "Motor Warning "/1 -> Fault Code Determination/4(EM_Warning)
  Fault Code Determination/1(Fault_Code) -> Scope/3, "Fault Code "/1
  Bus Selector/2 -> Fault Code Determination/2(Battery_Temp), Scope/2  "<bcm_cell_tmax>"
  Ground/1 -> "CAN Communication Failures "/1(In1)
  "CAN Communication Failures "/1(Out1) -> Terminator/1
  Step/1 -> Mode Overide/2
  Constant1/1 -> ?
  Bus Selector/3 -> "Inverter Temp Selection "/1(In1)  "<EM_CAN_Out>"
  "Inverter Temp Selection "/1(Out1) -> Fault Code Determination/3(Inverter_Temp)
  Bus Selector/4 -> Fault Code Determination/8(bcm_dis_buf)  "<bcm_dis_buf>"

== system EcoSIM3_P2_C2_WIP/Supervisory Controller/Subsystem ==
  In1 : Inport
  Bus Creator : BusCreator  Inputs=3
  Bus Creator1 : BusCreator  Inputs=1
  Bus Selector : BusSelector  OutputSignals=ESS_Transmit.ESS_CAN_Out.BCM_Status.bcm_chgc_stat,ESS_Transmit.ESS_CAN_Out.BCM_Status.bcm_mainc_stat
  Constant : Constant
  Constant1 : Constant  Value=12.8
  Constant2 : Constant
  Constant3 : Constant  Value=0
  Logical Operator : Logic  Operator=OR  AllPortsSameDT=off  OutDataTypeStr=boolean
  Switch : Switch  Criteria=u2 > Threshold  Threshold=0.5
  Out1 : Outport
  wires:
  Switch/1 -> Bus Creator/1  "LowVoltEnblRq"
  Constant1/1 -> Bus Creator/2  "LwVltStpntCmnd"
  Constant2/1 -> Bus Creator/3  "PrplsnSysAtv"
  Bus Creator/1 -> Bus Creator1/1  "DC_DC"
  In1/1 -> Bus Selector/1
  Constant/1 -> Switch/1  "LowVoltEnablRq"
  Bus Selector/1 -> Logical Operator/1  "<bcm_chgc_stat>"
  Bus Selector/2 -> Logical Operator/2  "<bcm_mainc_stat>"
  Logical Operator/1 -> Switch/2
  Constant3/1 -> Switch/3
  Bus Creator1/1 -> Out1/1  "Non_Propulsion"

== system EcoSIM3_P2_C2_WIP/Supervisory Controller/Supervisory_IO ==
  note: 1) Add Subsystem or Model blocks as valid variant choices.
      | 2) You cannot connect blocks at this level. At simulation, connectivity is automatically
      | determined, based on the active variant and port name matching.
  From_Goto : Subsystem  VariantControl=Sim_type == 1
  VNT Kvaser : Subsystem  VariantControl=Sim_type == 3
  VNT Vector : Subsystem  VariantControl=Sim_type == 2

== system EcoSIM3_P2_C2_WIP/Driver/GM_Transmit/WheelTickLD ==
  In1 : Inport
  Constant : Constant  Value=360
  Constant1 : Constant  Value=1024
  Gain : Gain  Gain=360/(2*pi)
  Gain1 : Gain  Gain=49/360
  Math Function : Math  Operator=rem  SaturateOnIntegerOverflow=on
  Rounding Function1 : Rounding
  Scope : Scope
      settings: SaveName=ScopeData9
  Scope1 : Scope
      settings: SaveName=ScopeData14
  Out1 : Outport
  wires:
  Rounding Function1/1 -> Scope/1, Out1/1  "WRSLDWhlDistPlsCntr"
  In1/1 -> Scope1/1, Gain/1
  Constant1/1 -> Math Function/2
  Gain/1 -> Gain1/1
  Gain1/1 -> Math Function/1
  Math Function/1 -> Rounding Function1/1

== system EcoSIM3_P2_C2_WIP/Driver/GM_Transmit/WheelTickLND ==
  In1 : Inport
  Constant : Constant  Value=360
  Constant1 : Constant  Value=1024
  Gain : Gain  Gain=360/(2*pi)
  Gain1 : Gain  Gain=49/360
  Math Function : Math  Operator=rem  SaturateOnIntegerOverflow=on
  Rounding Function1 : Rounding
  Scope : Scope
      settings: SaveName=ScopeData9
  Scope1 : Scope
      settings: SaveName=ScopeData14
  Out1 : Outport
  wires:
  Math Function/1 -> Rounding Function1/1
  Gain1/1 -> Math Function/1
  Gain/1 -> Gain1/1
  Constant1/1 -> Math Function/2
  In1/1 -> Gain/1, Scope1/1
  Rounding Function1/1 -> Out1/1, Scope/1  "WRSLNDWhlDistPCntr"

== system EcoSIM3_P2_C2_WIP/Driver/GM_Transmit/WheelTickRD ==
  In1 : Inport
  Constant : Constant  Value=360
  Constant1 : Constant  Value=1024
  Gain : Gain  Gain=360/(2*pi)
  Gain1 : Gain  Gain=49/360
  Math Function : Math  Operator=rem  SaturateOnIntegerOverflow=on
  Rounding Function1 : Rounding
  Scope : Scope
      settings: SaveName=ScopeData9
  Scope1 : Scope
      settings: SaveName=ScopeData14
  Out1 : Outport
  wires:
  Math Function/1 -> Rounding Function1/1
  Gain1/1 -> Math Function/1
  Gain/1 -> Gain1/1
  Constant1/1 -> Math Function/2
  In1/1 -> Gain/1, Scope1/1
  Rounding Function1/1 -> Out1/1, Scope/1  "WRSRDWhlDistPlsCntr"

== system EcoSIM3_P2_C2_WIP/Driver/GM_Transmit/WheelTickRND ==
  In1 : Inport
  Constant : Constant  Value=360
  Constant1 : Constant  Value=1024
  Gain : Gain  Gain=360/(2*pi)
  Gain1 : Gain  Gain=49/360
  Math Function : Math  Operator=rem  SaturateOnIntegerOverflow=on
  Rounding Function1 : Rounding
  Scope : Scope
      settings: SaveName=ScopeData9
  Scope1 : Scope
      settings: SaveName=ScopeData14
  Out1 : Outport
  wires:
  Rounding Function1/1 -> Scope/1, Out1/1  "WRSRNDWhlDistPCntr"
  In1/1 -> Scope1/1, Gain/1
  Constant1/1 -> Math Function/2
  Gain/1 -> Gain1/1
  Gain1/1 -> Math Function/1
  Math Function/1 -> Rounding Function1/1

== system EcoSIM3_P2_C2_WIP/Driver/PI Controller/Delay ==
  Velocity_Profile [m/s] : Inport
  Transfer Fcn1 : TransferFcn  Denominator=[1 1]
  Transport Delay : TransportDelay  Commented=on  DelayTime=0
  Pre_Velocity_Profile [m/s] : Outport
  wires:
  Transfer Fcn1/1 -> Pre_Velocity_Profile [m/s]/1
  Velocity_Profile [m/s]/1 -> Transfer Fcn1/1

== system EcoSIM3_P2_C2_WIP/Driver/PI Controller/Dyno Data Variant ==
  note: 1) Add Subsystem or Model blocks as valid variant choices.
      | 2) You cannot connect blocks at this level. At simulation, connectivity is automatically
      | determined, based on the active variant and port name matching.
  AcclnTest250 : Subsystem  VariantControl=Comparison_Acceleration
  Coastdown : Subsystem  VariantControl=Comparison_Coastdown
  HWFET_150 : Subsystem  VariantControl=Comparison_HWFET
  US06_150 : Subsystem  VariantControl=Comparison_US06
  Alpha : Outport
  Beta : Outport  Port=2

== system EcoSIM3_P2_C2_WIP/Driver/Startup Dummy/Vehicle Start ==
  PRNDL : Inport
  Key Pos : Inport  Port=2
  Brake_Position : Inport  Port=3
  Chart1 : Stateflow chart  TreatAsAtomicUnit=on
  Compare To Constant : simulink/Logic and Bit Operations/Compare To Constant  relop===  const=1  OutDataTypeStr=boolean
  Compare To Constant1 : simulink/Logic and Bit Operations/Compare To Constant  relop=>=  const=5  OutDataTypeStr=boolean
  Logical Operator2 : Logic  AllPortsSameDT=off  OutDataTypeStr=boolean
  Park_check : Stateflow chart  TreatAsAtomicUnit=on
  Percent_brake : Constant  Value=20
  Step : Step  Time=2  Before=1  After=0  SampleTime=0
  Switch : Switch  Criteria=u2 > Threshold  Threshold=0.5
  Key State : Outport
  SysPwrMd : Outport  Port=2
  Brake Position : Outport  Port=3
  wires:
  PRNDL/1 -> Park_check/1(p_in)
  Key Pos/1 -> Chart1/1(Push_Button)
  Compare To Constant/1 -> Logical Operator2/1
  Compare To Constant1/1 -> Logical Operator2/2
  Switch/1 -> Park_check/2(beta), Compare To Constant1/1, Brake Position/1  "BrkPdlPos"
  Step/1 -> Switch/2
  Percent_brake/1 -> Switch/1
  Brake_Position/1 -> Switch/3
  Logical Operator2/1 -> Chart1/2(Brk_PRNDL)
  Chart1/2(SysPwrMd) -> SysPwrMd/1
  Chart1/1(Key_State) -> Key State/1  "Accessory_Wake"
  Park_check/1(position) -> Compare To Constant/1  "PRNDL_position"

== system EcoSIM3_P2_C2_WIP/GCM/GCM_IO/From_Goto ==
  Bus Creator : BusCreator
  Bus Selector : BusSelector  OutputSignals=GCM_CAN_Out,GCM_Electrical_Out  OutputAsBus=on
  Bus Selector1 : BusSelector  OutputSignals=GM_Transmit,Brusa_Transmit,Mastershift_Transmit
  Bus Selector2 : BusSelector  OutputSignals=Supervisory_Requests.Supervisory_CAN.GCM_Messages_Transmission
  tag scope: From_GCM=global, GCM_from_CAN=global
  wires:
  Bus Creator/1 -> [GCM_from_CAN]
  [GCM_To_CAN] -> Bus Selector/1
  Bus Selector/1 -> [From_GCM]  "From_GCM"
  [From_ECUs] -> Bus Selector1/1
  Bus Selector1/1 -> Bus Creator/1  "<GM_Transmit>"
  Bus Selector1/2 -> Bus Creator/2  "<Brusa_Transmit>"
  [From_Supervisory] -> Bus Selector2/1
  Bus Selector2/1 -> Bus Creator/4  "<GCM_Messages_Transmission>"
  Bus Selector1/3 -> Bus Creator/3  "<Mastershift_Transmit>"

== system EcoSIM3_P2_C2_WIP/GCM/GCM_IO/VNT Kvaser ==
  CAN Rx : Subsystem
  CAN Tx : Subsystem
  Electrical Rx : Subsystem
  Electrical Tx : Subsystem
  Spine : Subsystem
  wires:
  Spine/1(Electrical Tx) -> Electrical Tx/1(Electrical)
  Spine/2(CAN Tx) -> CAN Tx/1(CAN)
  Electrical Rx/1(Electrical) -> Spine/1(Electrical Rx)
  CAN Rx/1(CAN) -> Spine/2(CAN Rx)

== system EcoSIM3_P2_C2_WIP/GCM/GCM_IO/VNT Vector ==
  CAN Rx : Subsystem
  CAN Tx : Subsystem
  Electrical Rx : Subsystem
  Electrical Tx : Subsystem
  Spine : Subsystem
  wires:
  Spine/1(Electrical Tx) -> Electrical Tx/1(Electrical)
  Spine/2(CAN Tx) -> CAN Tx/1(CAN)
  Electrical Rx/1(Electrical) -> Spine/1(Electrical Rx)
  CAN Rx/1(CAN) -> Spine/2(CAN Rx)

== system EcoSIM3_P2_C2_WIP/GCM/ProcessMode/MastershiftMessages ==
  Inputs : Inport
  Add : Sum  Inputs=+-
  Bus Creator : BusCreator  Inputs=3
  Bus Creator1 : BusCreator  Inputs=2
  Bus Selector : BusSelector  OutputSignals=GCM_Messages_Transmission.GCM_Gear_Request,GCM_Messages_Transmission.Clutch_Status,Mastershift_Transmit.Mastershift_Electrical_Out.Mastershift_Gear
  Display : Display
  Display1 : Display
  Display2 : Display
  Memory : Memory
  Memory1 : Memory  X0=1
  Mux : Mux  Inputs=2
  Rounding Function : Rounding  Operator=round
  Scope : Scope
      settings: SaveName=ScopeData27
  Scope1 : Scope
      settings: SaveName=ScopeData34
  Scope2 : Scope  NumInputPorts=2
      settings: YMin=-5~-5  YMax=5~5  SaveName=ScopeData44
  Scope3 : Scope  NumInputPorts=3
      settings: YMin=-5~-5~-5  YMax=5~5~5  SaveName=ScopeData46
  Scope4 : Scope  NumInputPorts=2
      settings: YMin=-5~-5  YMax=5~5  SaveName=ScopeData47
  Scope5 : Scope
      settings: SaveName=ScopeData62
  Shift Signal Generator : Stateflow chart  TreatAsAtomicUnit=on
  To Workspace : ToWorkspace  VariableName=defectivevalue  SampleTime=-1
  MShift : Outport
  MABx : Outport  Port=2
  wires:
  Inputs/1 -> Bus Selector/1
  Shift Signal Generator/1(Upshift_Sw) -> Bus Creator/1, Scope2/1  "Upshift_Sw"
  Shift Signal Generator/2(Downshift_Sw) -> Scope2/2, Bus Creator/2  "Downshift_Sw"
  Bus Selector/1 -> Add/2, Display/1, Rounding Function/1, Mux/2  "<GCM_Gear_Request>"
  Bus Creator/1 -> MShift/1  "Mastershift_Messages"
  Bus Selector/2 -> Shift Signal Generator/2(Clutch_Status)  "<Clutch_Status>"
  Shift Signal Generator/3(Clutch_Sw) -> Bus Creator/3  "Clutch_Sw"
  Memory1/1 -> Bus Creator1/1  "Shift_Complete"
  Bus Creator1/1 -> MABx/1  "Shift_Status_to_MABx"
  Bus Selector/3 -> Memory/1  "<Mastershift_Gear>"
  Shift Signal Generator/7(Shift_Complete) -> Scope4/1, Memory1/1  "Shift_Complete"
  Shift Signal Generator/4(Local_Count) -> Scope3/1
  Shift Signal Generator/5(Shift_Count) -> Display2/1, Scope3/2
  Shift Signal Generator/6(state) -> Scope3/3
  Rounding Function/1 -> Shift Signal Generator/1(GCM_Gear_Request), Add/1, Mux/1
  Mux/1 -> Scope1/1
  Add/1 -> Scope5/1, To Workspace/1
  Memory/1 -> Display1/1, Bus Creator1/2, Scope4/2, Scope/1, Shift Signal Generator/3(Gear_From_Mastershift)  "GCM_Reported_Gear"

== system EcoSIM3_P2_C2_WIP/Model Parameters/Drive Cycle Selection/Demo Cycle ==
  Compare To Constant : simulink/Logic and Bit Operations/Compare To Constant  relop=>=  const=24.5  OutDataTypeStr=boolean
  Constant : Constant  Value=24.5872
  Ramp : simulink/Sources/Ramp  slope=24.5872/10  start=5  X0=0
  Switch : Switch  Criteria=u2 > Threshold
  v : Outport
  wires:
  Switch/1 -> v/1
  Constant/1 -> Switch/1
  Ramp/1 -> Switch/3, Compare To Constant/1
  Compare To Constant/1 -> Switch/2

== system EcoSIM3_P2_C2_WIP/Powertrain/Accessories Power Module/CAN_Receive ==
  Bus Creator : BusCreator  Inputs=2
  Bus Creator1 : BusCreator  Inputs=1
  Bus Creator2 : BusCreator  Inputs=5
  Bus Creator4 : BusCreator  Inputs=2
  Constant5 : Constant  Value=2
  Constant6 : Constant
  Ramp : simulink/Sources/Ramp  slope=2  start=0  X0=0
  Ramp1 : simulink/Sources/Ramp  slope=10  start=0  X0=20
  Ramp2 : simulink/Sources/Ramp  slope=2  start=0  X0=100
  Signal Builder : Subsystem  Tag=STV Subsys  LoadFcn=sigbuilder_block('load');  StartFcn=sigbuilder_block('start');  StopFcn=sigbuilder_block('stop');  ClipboardFcn=sigbuilder_block('clipboard');  mask(Sigbuilder block){}
      mask help: Simulink:masks:SigbuilderBlock_MD
      mask init:
      | if ~strcmp(get_param(bdroot(gcbh),'SimulationStatus'),'stopped') tuvar = sigbuilder_block('maskInit'); end
      settings: CopyFcn=sigbuilder_block('copy');  DeleteFcn=sigbuilder_block('delete');  ModelCloseFcn=sigbuilder_block('modelClose');  PreSaveFcn=sigbuilder_block('preSave');  PauseFcn=sigbuilder_block('pause');  ContinueFcn=sigbuilder_block('continue');  NameChangeFcn=sigbuilder_block('namechange');  OpenFcn=sigbuilder_block('open',[437.6 199.2 550.4 400 ]);  CloseFcn=sigbuilder_block('close');
      mask Display: plot(0, 0, 100, 100,[2, 2, 32, 32, 2], [68, 8, 8, 68, 68],[32, 2], [38, 38], [32, 19, 2],[53, 60, 44], [32, 17, 17, 2],[16, 16, 31, 31]);txt = getActiveGroup(gcbh);text(2, 100, txt,'verticalAlignment', 'top');
  Switch : Switch  Criteria=u2 > Threshold
  From_CAN : Outport
  wires:
  Signal Builder/3(Signal 4) -> Switch/1
  Constant5/1 -> Switch/3
  Constant6/1 -> Switch/2
  Bus Creator2/1 -> Bus Creator4/2  "CAN Signal"
  Bus Creator1/1 -> Bus Creator4/1  "Electrical Signal"
  Signal Builder/1(Signal 1) -> Bus Creator1/1  "PowerUp"
  Ramp1/1 -> Bus Creator2/5  "PowerReq"
  Signal Builder/2(Signal 2) -> Bus Creator2/1  "BCMMainCStart"
  Switch/1 -> Bus Creator2/2  "LowVoltEnblRq"
  Ramp/1 -> Bus Creator2/3  "LwVltStpntCmnd"
  Ramp2/1 -> Bus Creator2/4  "bcmVbat"
  [DCDC_SoftECU_Receive] -> Bus Creator/1  "DCDC_SoftECU_Receive"
  [ESS_SoftECU_Transmit] -> Bus Creator/2
  Bus Creator/1 -> From_CAN/1

== system EcoSIM3_P2_C2_WIP/Powertrain/Accessories Power Module/CAN_Transmit ==
  To_CAN : Inport
  Bus Creator : BusCreator  Inputs=2
  Bus Creator1 : BusCreator  Inputs=2
  Ground : Ground
  Ground1 : Ground
  tag scope: DCDC_SoftECU_Transmit=global
  wires:
  Ground1/1 -> Bus Creator1/2  "Dummy2"
  Ground/1 -> Bus Creator1/1  "Dummy1"
  Bus Creator1/1 -> Bus Creator/2  "APM_Electrical_Out"
  To_CAN/1 -> Bus Creator/1
  Bus Creator/1 -> [DCDC_SoftECU_Transmit]  "DCDC_Transmit"

== system EcoSIM3_P2_C2_WIP/Powertrain/Accessories Power Module/Component Power ==
  Add : Sum
  Bus Selector : BusSelector  OutputSignals=ESS_CAN_Out.BCM_Status.bcm_vbat
  Bus Selector1 : BusSelector  OutputSignals=Veh_Plugged_In
  Bus Selector2 : BusSelector  OutputSignals=DCDC_CAN.PTEI_Hybrid_General_Status_1.LowVoltEnblRq
  Constant : Constant
  Constant1 : Constant  Value=12
  Constant2 : Constant  Value=28
  Constant3 : Constant  Value=30
  Constant4 : Constant  Value=4.41
  Constant5 : Constant  Value=0
  Constant6 : Constant  Value=0
  DCDC Dyno avg : Constant  Value=1.7
  DCDC avg current_A : Constant  Value=1.7918
  Ground : Ground
  HVAC : Subsystem
  Memory : Memory
  Parameters : Subsystem
  Product : Product
  Switch : Switch  Criteria=u2 > Threshold  Threshold=0.5
  Switch1 : Switch  Criteria=u2 > Threshold  Threshold=0.5
  Terminator : Terminator
  The Corrupter : Subsystem
  Out2 : Outport
  wires:
  Switch1/1 -> Out2/1  "Accessories_Power_In_W"
  Add/1 -> Switch/3  "Accessories_Power_In_W"
  Parameters/1(P) -> The Corrupter/2(Noise Parameters)
  Constant4/1 -> HVAC/5(Current)
  [Simulation_Parameters] -> Bus Selector1/1
  Constant5/1 -> Switch/1
  Product/1 -> Add/2
  [ESS_SoftECU_Transmit] -> Bus Selector/1
  Constant/1 -> HVAC/1(AC_Mode)
  Constant2/1 -> HVAC/3(AC_Engagement_pressure)
  [DCDC_SoftECU_Receive] -> Bus Selector2/1
  Bus Selector2/1 -> Switch1/2  "<LowVoltEnblRq>"
  DCDC avg current_A/1 -> The Corrupter/1(Signal In)
  HVAC/1(HVAC Pwr_W) -> Add/1
  Ground/1 -> Terminator/1
  Memory/1 -> HVAC/6(Voltage), Product/2
  Constant1/1 -> HVAC/2(AC_Press_bar)
  Bus Selector/1 -> Memory/1  "<bcm_vbat>"
  Constant3/1 -> HVAC/4(AC_max_pressure)
  DCDC Dyno avg/1 -> Product/1  "APM_Current"
  Switch/1 -> Switch1/1
  Bus Selector1/1 -> Switch/2  "<Veh_Plugged_In>"
  Constant6/1 -> Switch1/3
